simulink model "w3prob2"  (R2020a)
settings: Solver=VariableStepAuto  StartTime=0.0  StopTime=10.0  RelTol=1e-3
settings Model: Creator=Anjali123  LastModifiedBy=Anjali123

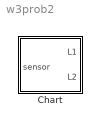
== system w3prob2 ==
  Chart : Stateflow chart  TreatAsAtomicUnit=on

== stateflow chart w3prob2/Chart ==
  settings: stateMachineType=MOORE_MACHINE
  state Stop_to_Go
    L1 = RED;
    L2 = YELLOW;
  state Stop
    L1 = RED;
    L2 = GREEN;
  state Stop_for_Traffic
    L1 = RED;
    L2 = GREEN;
  state Go
    L1 = GREEN;
    L2 = RED;
  state Go_to_Stop
    L1 = YELLOW;
    L2 = RED;
  (default) -> Stop
  Stop_for_Traffic -> Stop_to_Go : [sensor]
  Stop -> Stop_for_Traffic : after(20,tick)
  Stop_to_Go -> Go : after(3,tick)
  Go_to_Stop -> Stop : after(3,tick)
  Go -> Go_to_Stop : after(10,tick)
  data: sensor input; L1 output; L2 output; GREEN constant double =2; RED constant double =0; YELLOW constant double =1
